simulink model "lab_modulation_am_sync_det"  (R2025a)
settings: Solver=VariableStepAuto  StartTime=0.0  StopTime=1  RelTol=1e-3
libraries: dspfdesign x2
settings Model: Creator=Ksenia Kochneva  LastModifiedBy=Ksenia Kochneva

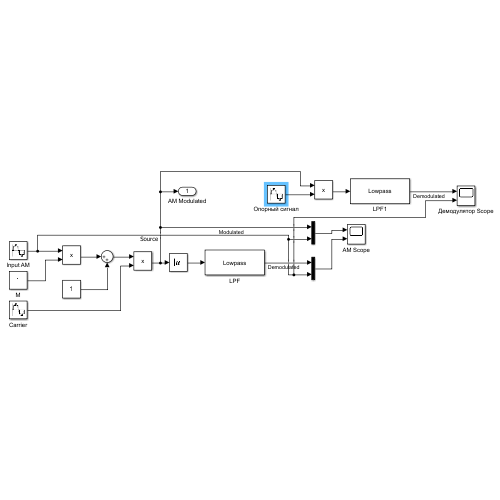
[thumbnail: Simulink's stored preview of the top-level diagram]
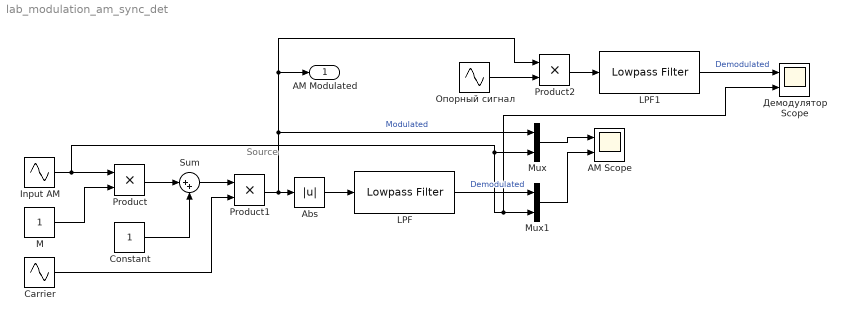
== system lab_modulation_am_sync_det ==
  note: Source
  AM Scope : Scope  NumInputPorts=2
      settings: ActiveDisplayYMinimum=-1  ActiveDisplayYMaximum=1
  Abs : Abs  SaturateOnIntegerOverflow=off
  Carrier : Sin  Frequency=100*2*pi  SampleTime=0.0001
  Constant : Constant
  Input AM : Sin  Frequency=2*2*pi  SampleTime=0.0001
  LPF : dspfdesign/Lowpass Filter  FilterType=FIR  DesignForMinimumOrder=on  FilterOrder=50  PassbandFrequency=0.1  StopbandFrequency=100  PassbandRipple=0.1  StopbandAttenuation=80  SampleRate=44100  SimulateUsing=Interpreted execution  roundingMode=Floor  coeffsDataTypeStr=fixdt(1,16)
  LPF1 : dspfdesign/Lowpass Filter  FilterType=FIR  DesignForMinimumOrder=on  FilterOrder=50  PassbandFrequency=10  StopbandFrequency=100  PassbandRipple=0.1  StopbandAttenuation=80  SampleRate=44100  SimulateUsing=Interpreted execution  roundingMode=Floor  coeffsDataTypeStr=fixdt(1,16)
  M : Constant
  Mux : Mux  Inputs=2
  Mux1 : Mux  Inputs=2
  Product : Product
  Product1 : Product
  Product2 : Product
  Sum : Sum  Inputs=|++
  Демодулятор Scope : Scope  NumInputPorts=2
      settings: ActiveDisplayYMinimum=-1.2499999999998153  ActiveDisplayYMaximum=1.2499999999999212
  Опорный сигнал : Sin  Frequency=100*2*pi  SampleTime=0.0001
  AM Modulated : Outport
  wires:
  Product/1 -> Sum/1
  Constant/1 -> Sum/2
  Product1/1 -> Product2/1, AM Modulated/1, Mux/1, Abs/1  "Modulated"
  Abs/1 -> LPF/1
  LPF/1 -> Mux1/1  "Demodulated"
  M/1 -> Product/2
  Input AM/1 -> Mux/2, Демодулятор Scope/2, Mux1/2, Product/1
  Sum/1 -> Product1/1
  Carrier/1 -> Product1/2
  Mux/1 -> AM Scope/1
  Mux1/1 -> AM Scope/2
  Опорный сигнал/1 -> Product2/2
  Product2/1 -> LPF1/1
  LPF1/1 -> Демодулятор Scope/1  "Demodulated"
